simulink model "TwoBatteriesMonitor"  (Simulink 7.4)
settings: Solver=ode45  StartTime=0.0  StopTime=10.0  RelTol=1e-3
settings Model: Creator=Andre  LastModifiedBy=Andre

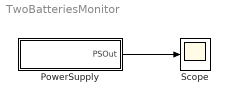
== system TwoBatteriesMonitor ==
  PowerSupply : Subsystem
  Scope : Scope
  wires:
  PowerSupply/1(PSOut) -> Scope/1

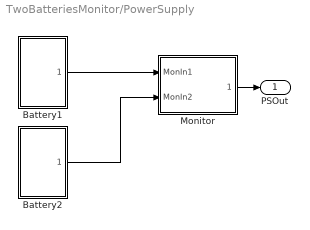
== system TwoBatteriesMonitor/PowerSupply ==
  Battery1 : Subsystem  mask{voltage=5, chargedTime=3}
      mask prompts: voltage "Battery voltage"; chargedTime "Charged time"
  Battery2 : Subsystem  mask{voltage=5, chargedTime=3}
      mask prompts: voltage "Battery voltage"; chargedTime "Charged time"
  Monitor : Subsystem  mask{threshold=3}
      mask prompts: threshold "Highlow threshold"
      mask init:
      | 3
  PSOut : Outport
  wires:
  Battery2/1(BatOut1) -> Monitor/2(MonIn2)
  Battery1/1(BatOut1) -> Monitor/1(MonIn1)
  Monitor/1(MonOut) -> PSOut/1

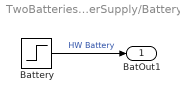
== system TwoBatteriesMonitor/PowerSupply/Battery1 ==
  Battery : Step  Time=chargedTime  Before=5  After=0  SampleTime=1
  BatOut1 : Outport  OutDataType=fixdt(1, 16)  OutScaling=2^0
  wires:
  Battery/1 -> BatOut1/1  "HW Battery"

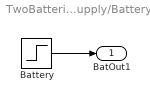
== system TwoBatteriesMonitor/PowerSupply/Battery2 ==
  Battery : Step  Time=chargedTime  Before=5  After=0  SampleTime=1
  BatOut1 : Outport  OutDataType=fixdt(1, 16)  OutScaling=2^0
  wires:
  Battery/1 -> BatOut1/1

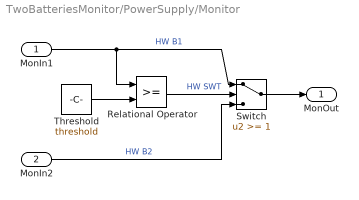
== system TwoBatteriesMonitor/PowerSupply/Monitor ==
  MonIn1 : Inport
  MonIn2 : Inport  Port=2
  Relational Operator : RelationalOperator  LogicOutDataTypeMode=boolean  LogicDataType=fixdt(0, 8)  OutDataTypeStr=boolean
  Switch : Switch  Threshold=1  OutDataType=fixdt(1, 16)  OutScaling=2^0
  Threshold : Constant  Value=threshold  OutDataType=fixdt(1, 16)  OutScaling=2^0
  MonOut : Outport
  wires:
  MonIn1/1 -> Relational Operator/1, Switch/1  "HW B1"
  Relational Operator/1 -> Switch/2  "HW SWT"
  Switch/1 -> MonOut/1
  MonIn2/1 -> Switch/3  "HW B2"
  Threshold/1 -> Relational Operator/2
